simulink model "optsim"  (Simulink 7.6)
settings: Solver=ode5  SolverMode=SingleTasking  StartTime=0.0  StopTime=100  FixedStep=1  RelTol=1e-3  AbsTol=1e-6
PreLoadFcn:
  | a1=3; a2=43;
PostLoadFcn:
  | optsiminit
values from neighbouring files (symbols this model uses):
  D = 2    [ParabGa.m]    (also in PidGa.m = 3; expoGa.m)
  Kd = x(3)    [PidGa.m]    (also in optsiminit.m = 1.9688; tracklsq.m = pid(3))
  Ki = x(2)    [PidGa.m]    (also in optsiminit.m = 0.0504; tracklsq.m = pid(2))
  Kp = x(1)    [PidGa.m]    (also in optsiminit.m = 0.63; tracklsq.m = pid(1))
undefined symbols (not defined in the file or in its folder): I
settings Model: Creator=nikita  LastModifiedBy=miguel  ExtModeTrigMode=oneshot  ExtModeArmWhenConnect=off
settings DataIOCC: LimitDataPoints=off  SaveTime=off  StateSaveName=x  TimeSaveName=t
settings OptimizationCC: BooleanDataType=off  InitFltsAndDblsToZero=on
settings DebuggingCC: SaveWithParameterizedLinksMsg=none  SignalResolutionControl=TryResolveAllWithWarning  SolverPrmCheckMsg=none  MultiTaskDSMMsg=warning  MultiTaskCondExecSysMsg=none  IntegerOverflowMsg=none  StrictBusMsg=None
settings HardwareCC: TargetUnknown=on
settings RTWCC: IncludeERTFirstTime=on
settings GRTTargetCC: TargetFcnLib=ansi_tfl_tmw.mat

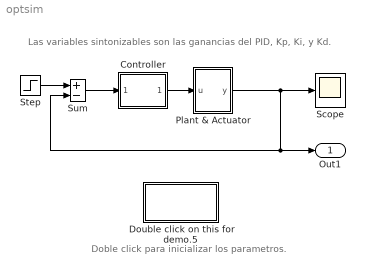
== system optsim ==
  note: Doble click para inicializar los parametros.
  note: Las variables sintonizables son las ganancias del PID, Kp, Ki, y Kd.
  Controller : Subsystem  mask(PID Controller){P=Kp,  I=Ki,  D=Kd}
      mask prompts: P "Proportional:";  I "Integral";  D "Derivative:"
      mask help: Enter expressions for proportional, integral, and derivative terms.
      mask Help: This block implements a PID controller where paramaters are entered for the Proportional, Integral and Derivative terms.
      mask Display: disp('PID')
  Double click on this for demo.5 : Subsystem
      settings: OpenFcn=optsiminit
      mask Display: disp('optsiminit')
  Plant & Actuator : Subsystem
  Scope : Scope
      settings: TickLabels=on  TimeRange=100  YMin=0  YMax=1.4
  Step : Step  Time=0  SampleTime=0
  Sum : Sum  Inputs=+-  SaturateOnIntegerOverflow=on  InputSameDT=on  OutDataTypeStr=Inherit: Same as first input
  Out1 : Outport
  wires:
  Plant & Actuator/1(y) -> Sum/2, Out1/1, Scope/1
  Sum/1 -> Controller/1(In_1)
  Step/1 -> Sum/1
  Controller/1(Out_1) -> Plant & Actuator/1("u ")

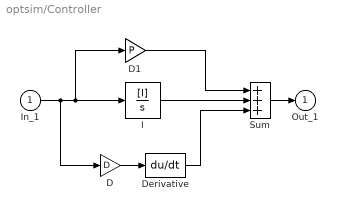
== system optsim/Controller ==
  In_1 : Inport
  D : Gain  Gain=D  SaturateOnIntegerOverflow=on  OutDataTypeStr=Inherit: Same as input  ParamDataTypeStr=Inherit: Same as input
  D1 : Gain  Gain=P  SaturateOnIntegerOverflow=on  OutDataTypeStr=Inherit: Same as input  ParamDataTypeStr=Inherit: Same as input
  Derivative : Derivative
  I : TransferFcn  Numerator=[I]  Denominator=[1 0]
  Sum : Sum  Inputs=+++  SaturateOnIntegerOverflow=on  InputSameDT=on  OutDataTypeStr=Inherit: Same as first input
  Out_1 : Outport  InitialOutput=0
  wires:
  In_1/1 -> D1/1, I/1, D/1
  Sum/1 -> Out_1/1
  D/1 -> Derivative/1
  Derivative/1 -> Sum/3
  I/1 -> Sum/2
  D1/1 -> Sum/1

== system optsim/Double click on this for demo.5 ==

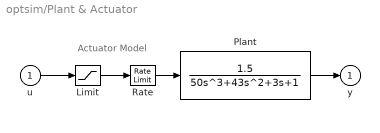
== system optsim/Plant & Actuator ==
  note: Actuator Model
  "u " : Inport
  Limit : Saturate  UpperLimit=2  LowerLimit=-2
  Plant : TransferFcn  Numerator=[1.5]  Denominator=[50 43 3 1]
  Rate : RateLimiter  RisingSlewLimit=0.8  FallingSlewLimit=-0.8
  y : Outport  InitialOutput=0
  wires:
  Plant/1 -> y/1
  "u "/1 -> Limit/1
  Rate/1 -> Plant/1
  Limit/1 -> Rate/1
